simulink model "verify_create_EB_mdl"  (R2018b)
settings: Solver=FixedStepDiscrete  StartTime=0.0  StopTime=10.0  FixedStep=0.5  RelTol=1e-3
libraries: simulink x2, carnot x1
settings Model: Creator=P41573  LastModifiedBy=drhf
settings DataIOCC: SaveFormat=Array  SignalLogging=off
settings SFSimCC: SimUseLocalCustomCode=off
settings RTWCC: RTWUseLocalCustomCode=off
settings CodeAppCC: StateflowObjectComments=on

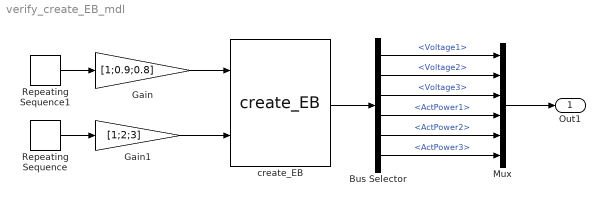
== system verify_create_EB_mdl ==
  Bus Selector : BusSelector  OutputSignals=Voltage1,Voltage2,Voltage3,ActPower1,ActPower2,ActPower3
  Gain : Gain  Gain=[1;0.9;0.8]
  Gain1 : Gain  Gain=[1;2;3]
  Mux : Mux  Inputs=6
  Repeating Sequence : simulink/Sources/Repeating Sequence  rep_seq_t=[0 5 10]  rep_seq_y=[0 500 0]
  Repeating Sequence1 : simulink/Sources/Repeating Sequence  rep_seq_t=[0 5 10]  rep_seq_y=[220 240 220]
  create_EB : carnot/Source/Simple/create_EB  eID=AC_3P  f=50  pf1=1  pf2=1  pf3=1
  Out1 : Outport
  wires:
  Repeating Sequence1/1 -> Gain/1
  Repeating Sequence/1 -> Gain1/1
  Bus Selector/1 -> Mux/1  "<Voltage1>"
  Bus Selector/5 -> Mux/5  "<ActPower2>"
  Gain/1 -> create_EB/1
  Gain1/1 -> create_EB/2
  create_EB/1 -> Bus Selector/1
  Bus Selector/2 -> Mux/2  "<Voltage2>"
  Bus Selector/3 -> Mux/3  "<Voltage3>"
  Bus Selector/4 -> Mux/4  "<ActPower1>"
  Bus Selector/6 -> Mux/6  "<ActPower3>"
  Mux/1 -> Out1/1
